simulink model "randomControllerSimOLD"  (R2015a)
settings: Solver=ode45  StartTime=0.0  StopTime=1.5  FixedStep=1/10000  RelTol=1e-6
values from neighbouring files (symbols this model uses):
  B_f = 7.7e-3    (= 0.0077)    [discreteOfModel.m]    (also in randomController.m = 0.0074)
  B_w = 17.03e-6    (= 1.703e-05)    [discreteOfModel.m]    (also in randomController.m)
  g = 9.82    [discreteOfModel.m]    (also in randomController.m)
  J_f = 4.8e-3    (= 0.0048)    [discreteOfModel.m]    (also in randomController.m = 0.0056)
  J_w = 0.601e-3    (= 0.000601)    [discreteOfModel.m]    (also in randomController.m)
  l_f = 0.08498    [discreteOfModel.m]    (also in randomController.m)
  l_w = 0.093    [discreteOfModel.m]    (also in randomController.m)
  m_f = 0.77-m_w    (= 0.548)    [discreteOfModel.m]    (also in randomController.m)
  m_w = 0.222    [discreteOfModel.m]    (also in randomController.m)
settings Model: CovSFcnEnable=off  Creator=USUARIO  LastModifiedBy=USUARIO
settings DataIOCC: LimitDataPoints=off  SignalLoggingSaveFormat=ModelDataLogs
settings DebuggingCC: SolverPrmCheckMsg=warning

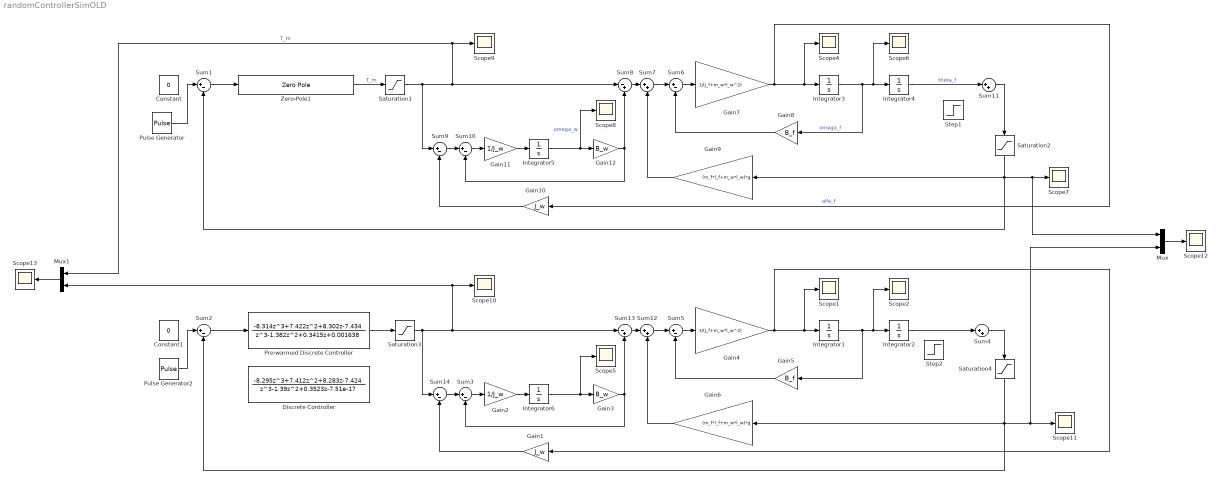
== system randomControllerSimOLD ==
  Constant : Constant  Value=0
  Constant1 : Constant  Value=0
  Discrete Controller : DiscreteTransferFcn  Numerator=[-8.295 7.412 8.283 -7.424]  Denominator=[1 -1.39 0.3523 -7.51e-17]  SampleTime=1/100
  Gain1 : Gain  Gain=J_w
  Gain10 : Gain  Gain=J_w
  Gain11 : Gain  Gain=1/J_w
  Gain12 : Gain  Gain=B_w
  Gain2 : Gain  Gain=1/J_w
  Gain3 : Gain  Gain=B_w
  Gain4 : Gain  Gain=1/(J_f+m_w*l_w^2)
  Gain5 : Gain  Gain=B_f
  Gain6 : Gain  Gain=(m_f*l_f+m_w*l_w)*g
  Gain7 : Gain  Gain=1/(J_f+m_w*l_w^2)
  Gain8 : Gain  Gain=B_f
  Gain9 : Gain  Gain=(m_f*l_f+m_w*l_w)*g
  Integrator{1..6} (6 alike) : Integrator
  Mux : Mux  Inputs=2
  Mux1 : Mux  Inputs=2
  Pre-warmed Discrete Controller : DiscreteTransferFcn  Numerator=[-8.314 7.422 8.302 -7.434]  Denominator=[1 -1.382 0.3415 0.001638]  SampleTime=1/100
  Pulse Generator : DiscretePulseGenerator  PulseType=Time based  Amplitude=-0.05  Period=10  PulseWidth=0.005
  Pulse Generator2 : DiscretePulseGenerator  PulseType=Time based  Amplitude=-0.05  Period=10  PulseWidth=0.005
  Saturation1 : Saturate  UpperLimit=4*0.0335  LowerLimit=-4*0.0335
  Saturation2 : Saturate  UpperLimit=0.85  LowerLimit=-0.72
  Saturation3 : Saturate  UpperLimit=4*0.0335  LowerLimit=-4*0.0335
  Saturation4 : Saturate  UpperLimit=0.85  LowerLimit=-0.72
  Scope{1..2,4..13} (12 alike) : Scope
      Scope1 settings: TimeRange=auto  LimitDataPoints=on  MaxDataPoints=5000  SaveToWorkspace=off  YMin=-43.84489  YMax=100.52539  SampleTime=-1
      Scope10 settings: TimeRange=auto  MaxDataPoints=5000  SaveToWorkspace=off  SaveName=ScopeData2  YMin=-0.00599  YMax=0.00528  SampleTime=-1
      Scope11 settings: TimeRange=auto  LimitDataPoints=on  MaxDataPoints=5000  SaveToWorkspace=off  YMin=-10  YMax=10  SampleTime=-1  DataFormat=Array
      Scope12 settings: TimeRange=2  MaxDataPoints=5000  SaveName=ScopeData2  YMin=-0.00804  YMax=0.00107  SampleTime=-1
      Scope13 settings: TimeRange=2  MaxDataPoints=5000  SaveName=ScopeData3  YMin=-0.1675  YMax=0.1675  SampleTime=-1
      Scope2 settings: TimeRange=auto  LimitDataPoints=on  MaxDataPoints=5000  SaveToWorkspace=off  SaveName=ScopeData3  YMin=-10  YMax=10  SampleTime=-1
      Scope4 settings: TimeRange=auto  LimitDataPoints=on  MaxDataPoints=5000  SaveToWorkspace=off  SaveName=ScopeData2  YMin=-10  YMax=10  SampleTime=-1
      Scope5 settings: TimeRange=auto  LimitDataPoints=on  MaxDataPoints=5000  SaveToWorkspace=off  SaveName=ScopeData5  YMin=-10  YMax=10  SampleTime=-1
      Scope6 settings: TimeRange=auto  LimitDataPoints=on  MaxDataPoints=5000  SaveToWorkspace=off  SaveName=ScopeData4  YMin=-10  YMax=10  SampleTime=-1
      Scope7 settings: TimeRange=2  MaxDataPoints=5000  SaveName=StepResponseData1  YMin=-0.000008  YMax=0.000003  SampleTime=-1
      Scope8 settings: TimeRange=auto  LimitDataPoints=on  MaxDataPoints=5000  SaveToWorkspace=off  SaveName=ScopeData6  YMin=-10  YMax=10  SampleTime=-1
      Scope9 settings: TimeRange=auto  LimitDataPoints=on  MaxDataPoints=5000  SaveToWorkspace=off  SaveName=ScopeData7  YMin=-0.00012  YMax=0.00046  SampleTime=-1
  Step1 : Step  Time=0.001  After=-0.0001  SampleTime=0
  Step2 : Step  Time=0.001  After=-0.0001  SampleTime=0
  Sum{1..3,5..6,9..10,14} (8 alike) : Sum  Inputs=|+-
  Sum{4,7,11..12} (4 alike) : Sum  Inputs=|++
  Sum13 : Sum  Inputs=|-+
  Sum8 : Sum  Inputs=|-+
  Zero-Pole1 : ZeroPole  Zeros=[-9.483 -1.599]  Poles=[-200 -100 5.539]  Gain=[-0.62737*200*100*5.539/9.483/1.599]
  wires:
  Gain7/1 -> Gain10/1, Scope4/1, Integrator3/1  "alfa_f"
  Integrator3/1 -> Gain8/1, Scope6/1, Integrator4/1  "omega_f"
  Sum6/1 -> Gain7/1
  Sum7/1 -> Sum6/1
  Gain8/1 -> Sum6/2
  Gain9/1 -> Sum7/2
  Sum8/1 -> Sum7/1
  Sum10/1 -> Gain11/1
  Gain11/1 -> Integrator5/1
  Gain10/1 -> Sum9/2
  Sum9/1 -> Sum10/1
  Integrator5/1 -> Scope8/1, Gain12/1  "omega_w"
  Gain12/1 -> Sum10/2, Sum8/2
  Zero-Pole1/1 -> Saturation1/1  "T_m"
  Integrator4/1 -> Sum11/1  "theta_f"
  Sum1/1 -> Zero-Pole1/1
  Sum11/1 -> Saturation2/1
  Saturation2/1 -> Scope7/1, Mux/1, Sum1/2, Gain9/1
  Saturation1/1 -> Sum8/1, Mux1/1, Scope9/1, Sum9/1  "T_m"
  Gain4/1 -> Gain1/1, Scope1/1, Integrator1/1
  Integrator1/1 -> Gain5/1, Scope2/1, Integrator2/1
  Sum5/1 -> Gain4/1
  Sum12/1 -> Sum5/1
  Gain5/1 -> Sum5/2
  Gain6/1 -> Sum12/2
  Sum13/1 -> Sum12/1
  Sum3/1 -> Gain2/1
  Gain2/1 -> Integrator6/1
  Gain1/1 -> Sum14/2
  Sum14/1 -> Sum3/1
  Integrator6/1 -> Scope5/1, Gain3/1
  Gain3/1 -> Sum3/2, Sum13/2
  Integrator2/1 -> Sum4/1
  Sum4/1 -> Saturation4/1
  Mux/1 -> Scope12/1
  Saturation3/1 -> Sum13/1, Scope10/1, Mux1/2, Sum14/1
  Mux1/1 -> Scope13/1
  Saturation4/1 -> Gain6/1, Sum2/2, Mux/2, Scope11/1
  Pulse Generator/1 -> Sum1/1
  Pulse Generator2/1 -> Sum2/1
  Pre-warmed Discrete Controller/1 -> Saturation3/1
  Sum2/1 -> Pre-warmed Discrete Controller/1
